simulink model "Bands7"  (R2018a)
settings: Solver=VariableStepAuto  StartTime=0.0  StopTime=0.01  RelTol=1e-3
undefined symbols (not defined in the file): fdesignblkfcn, G1, G2, G3, G4, G5, G6, G7, gcbh, get, T
libraries: dspsrcs4 x1, dspxfrm3 x1, dspobslib x1
(part 2 of 2)

== system Bands7/Filter Bank /Filter 5/Bandpass Filter ==
  In : Inport
  Generated Filter Block : DiscreteFir  Tag=BlockMethodSubSystem  Coefficients=[-9.58810852628409285e-08 2.32469628864830344e-08 3.86331465938965734e-07 -2.20783986023813804e-07 -1.02462161503425407e-06 9.81333351400442442e-07 2.09273408766862915e-06 -2.99371791475398828e-06 -3.31281199519531041e-06 7.28320341319092757e-06 3.72929278978732815e-06 -1.49118446680737189e-05 -1.28619054933032843e-06 2.64214782842553472e-05 -7.30535670538733667e-06 -4.08493754482887252e-05 2.62667010178946821e-05 5.4651471910311571e-05 -5.96059803468716439e-05 -6.08337254930435011e-05 0.000109152576803881542 4.90187993245668399e-05 -0.000171933793088775759 -6.98038786418440514e-06 0.000237712052040973639 -7.59195682598169175e-05 -0.000287739272451213301 0.000203714911831559986 0.000296061060386466359 -0.000368252612607931462 -0.000234224563044999241 0.000544966882564411012 7.94391823291172952e-05 -0.00069222980331757071 0.000175205090693047257 0.000756247105877000457 -0.000511177528820865924 -0.000682132059832164729 0.000879298715976650617 0.00042983022356125677 -0.00120235702500859549 8.77258524748186861e-06 0.00138752650373489021 -0.000596894132180304077 -0.00134769224831745205 0.00124972900223505501 0.00102741325130498683 -0.0018450930927680631 -0.000426327883119624086 0.00224817141909955257 -0.000388265080104680969 -0.00234590175869130949 0.00128635614321425968 0.00208214833483658449 -0.00209999739478021388 -0.00148249332143122895 0.00266396553918874521 0.000658647814734803546 -0.0028621525400130258 0.000212571742469404041 0.00266565875454846581 -0.000932999179653695786 -0.00214891728562074773 0.00133869642330399418 0.00147548828221558321 -0.00135067415892670063 -0.000854323950252250516 0.00100334938926574307 0.000477639688396269972 -0.000438719852644414991 -0.000459364165537671273 -0.000135265007016807301 0.000795224263203351232 0.000511214154350564083 -0.00136021337647840757 -0.000552719534013464326 0.00194748907395814056 0.000244187828567926819 -0.0023381878098927408 0.000299325687265161473 0.00237938988911029405 -0.000868808805288787903 -0.00204242142605657283 0.0012343976650798815 0.00143859817648006919 -0.00123031874608327089 -0.000783583969776330009 0.000820608820089682158 0.000320294511549712685 -0.000119378067820387741 -0.000226912149951525547 -0.000645229133491009355 0.00054439148237206338 0.00121327377293990388 -0.00115291167291446022 -0.00139256890304183235 0.00180982511450054396 0.00113764827880715857 -0.00223837184131480587 -0.00057554151761311117 0.00223549082946571023 -3.55594176082287081e-05 -0.0017570589557428162 0.000402862505289366588 0.00094481050398365421 -0.000315786849809520146 -8.00104639647764167e-05 -0.000262766749808934395 -0.000522506120992502206 0.00116955629342665774 0.000641039770527101907 -0.00209410080355902986 -0.000244184882697611556 0.00269575985622459886 -0.00048354262887346372 -0.00274133288650026249 0.00120335824971491267 0.00220797402718195517 -0.00155208512671623812 -0.00130634747033972379 0.00129152120570901786 0.000408549969613740665 -0.000416756600865931181 9.63079154092008047e-05 -0.000824671648667552309 3.58971676916477979e-05 0.00201744477211146089 -0.000791022589177617667 -0.00273938836172095673 0.00188315780959731355 0.00273707559579800235 -0.0028541270193768193 -0.00204361222754109468 0.00325286164607629588 0.000984752531566890094 -0.00282539339163617124 -6.22419908126786367e-05 0.00163636370351811513 -0.000245917406323728201 -6.56109702094782041e-05 -0.000309518401274032503 -0.00132835771435360172 0.00162485623429833338 0.00203067801396696491 -0.0032588688544591439 -0.00179094446626814697 0.00459217285623882837 0.000749014096506475657 -0.00507444040028377265 0.000594910613330368841 0.00446169817889733016 -0.00156551695937931826 -0.00294241174567129058 0.00158671475322137625 0.00109010796687163819 -0.000435806868879273497 0.000351161615849820692 -0.00163196222838977501 -0.000770829630763538625 0.00395176925736859426 -3.65997272116294625e-05 -0.00569705335793176636 0.00175038724886792969 0.00621616447243216168 -0.00361658993859075278 -0.00532206879955934506 ...(+7256 chars)]  InputProcessing=Columns as channels (frame based)
  Out : Outport
  wires:
  In/1 -> Generated Filter Block/1
  Generated Filter Block/1 -> Out/1

== system Bands7/Filter Bank /Filter 6/Bandpass Filter ==
  In : Inport
  Generated Filter Block : DiscreteFir  Tag=BlockMethodSubSystem  Coefficients=[-1.25255425151606446e-08 8.89638015557058461e-08 -1.00660481106791294e-07 -1.71542671618598763e-07 6.30727136722890552e-07 -4.94305586397416649e-07 -9.41860206286260817e-07 2.60648097200518803e-06 -1.51970142506445499e-06 -3.61925681579796005e-06 8.08811319906721527e-06 -3.49175116371090348e-06 -1.1058199124682812e-05 2.07298720252032752e-05 -6.26700739889994989e-06 -2.85833947368600613e-05 4.60081150553439048e-05 -8.46255439469102264e-06 -6.47651134006119471e-05 9.08836717492770435e-05 -6.44304383480617838e-06 -0.000131551007649326689 0.000162606489555876152 6.55019497498123363e-06 -0.000243150366983025702 0.000266628220200327355 4.05016863016043638e-05 -0.000413219537460888012 0.000404005983186840568 0.000107245375651426463 -0.000650375926198663683 0.000569142137305933137 0.000217148960754739669 -0.000952823316571735509 0.000748983248379460603 0.000374063015006662199 -0.00130367733422708963 0.000924651889340564049 0.000569711908969014187 -0.0016690706978893272 0.0010757723946409213 0.000779654225631718021 -0.0020009071412763371 0.00118658168412516052 0.000963374337522111194 -0.00224501117923517042 0.00125168654002985342 0.00107051093343472491 -0.00235353362539772676 0.00127864765455265052 0.00105348573675424209 -0.00229839700906786775 0.00128502102379148648 0.000884170524456743428 -0.00208118317329354348 0.00128930827508344026 0.000569581531915105055 -0.00173504472049494348 0.00129809096601209042 0.000160128275453357385 -0.0013163778185779477 0.00129442636713676066 -0.000255230684431742301 -0.000887736683498474154 0.0012339617878048127 -0.000569037034882513863 -0.000497533514369441661 0.00105396961220826767 -0.000687144670000418745 -0.000164654397395709356 0.000696271248643948572 -0.000563114550348206328 0.000124381414706665398 0.000138793139474224417 -0.000222564241775814856 0.000402274804298624654 -0.000575438119759497514 0.000234173942960876763 0.000695220164874023913 -0.00132582263997436381 0.000656595694415445445 0.000994957172509963652 -0.00192951581988383587 0.000891392271430931082 0.00124270486712862917 -0.0021872833289222687 0.000838066093421750095 0.00133698387209448617 -0.00195034211773934289 0.00049208229542788758 0.00116886917199326827 -0.00118712198309475531 -4.36832686119950414e-05 0.000675775510236198873 -2.33780320881614893e-05 -0.000588463769513059725 -0.000106648029153674808 0.00126649799565767924 -0.00094761156855736493 -0.00101986869618016056 0.00232436604491836115 -0.000988986407521479744 -0.00180479178356737335 0.00281579117468175495 -0.000701033724786980102 -0.00217461527176102034 0.00254679724689644074 -0.000205406431489680267 -0.00192000261778797233 0.001547055390059544 0.000286879953691100567 -0.00100959420040403879 8.29877302137138059e-05 0.000563205331859186072 0.000357732325524895325 -0.00141337049324328492 0.000506929173796110354 0.00178133273153402872 -0.00248238814787841468 0.000161355705397175963 0.00277292942611897294 -0.00279563684280270458 -0.000274283410010269879 0.00292624372174007724 -0.00227599204602179283 -0.000524851700467135474 0.00208324750860265986 -0.00112926975961976988 -0.000369102106795455838 0.000429435990301485981 0.000230803374986378014 0.000234616266742058391 -0.00153103119635096736 0.00134002527324787951 0.00108771505910517275 -0.00312742176945925415 0.00186306560293446419 0.00179669797102248734 -0.00375762732904636734 0.0017207113018726575 0.00192291441496002008 -0.00312251791732995982 0.00110854855834140132 0.00118620453962551154 -0.00136567096774006715 0.000394691550530183147 -0.000362156200121252611 0.000947076736786452091 -6.2252895142800825e-05 -0.00228292336609010622 0.00301487564500350436 -9.39968850170036242e-05 -0.00385680117783793576 0.00409449836575851833 0.000185135683972981641 -0.00433923981716520957 0.00378791711847140285 0.00042787366075095856 -0.00327610002517882571 0.00220736223664322849 0.000236086578017572434 -0.000753033868313336663 -5.73639565389522256e-05 -0.00060043166924552457 0.00254007828127078474 -0.00216656740971749983 ...(+7574 chars)]  InputProcessing=Columns as channels (frame based)
  Out : Outport
  wires:
  In/1 -> Generated Filter Block/1
  Generated Filter Block/1 -> Out/1

== system Bands7/Filter Bank /Filter 7/Bandpass Filter ==
  In : Inport
  Generated Filter Block : DiscreteFir  Tag=BlockMethodSubSystem  Coefficients=[1.73785777638198983e-08 5.53307655928696029e-08 -5.93261075754201142e-07 2.39151425515476142e-06 -6.48513630922282161e-06 1.34076757534754531e-05 -2.19514778171459608e-05 2.81125292022978393e-05 -2.54304009207347507e-05 7.77160995119231591e-06 2.56750310283883588e-05 -6.55244886674400545e-05 9.14386871994476703e-05 -7.89702444068962492e-05 1.38106561454960583e-05 9.2552034041583223e-05 -0.00019629525836815153 0.000233415676447405279 -0.000151571874020526014 -5.08961033605654563e-05 0.000302055501472180805 -0.000471848438432888762 0.000431172103111375027 -0.00013241288464823484 -0.000333224596582850524 0.000746513510533375097 -0.00085427096542935448 0.000512480179939020768 0.000197510427006736689 -0.000959758201500983009 0.00135473207975177678 -0.00108359599993431929 0.000169250182968863172 0.000993633909920033694 -0.00180012155352935171 0.00174972795567223316 -0.000751315472308702144 -0.000766187274657077343 0.00203186156748269 -0.00233241466939168932 0.00142321842761948514 0.000291081180231042168 -0.00193517820613313862 0.00262602239500718537 -0.00196835723958645008 0.000293868990911298408 0.00150845272728697389 -0.0024852883415886237 0.00215273227444568761 -0.000756876413467958624 -0.000891938083042786187 0.00190628271659362019 -0.00183031596807723611 0.000862643649298146676 0.000327866679015471245 -0.00105468168057194192 0.00103147230684341598 -0.000489843870350350065 -5.64931621242188649e-05 0.000213617305723943894 1.72764658636022303e-05 -0.000282287045395235141 0.000191187830209303781 0.000337066938522989266 -0.000967262286493930775 0.00117274045159026195 -0.000638002009766541018 -0.000456736720587986537 0.00149346411687726146 -0.00180136208817459689 0.00111384214709183229 0.00022266930227241171 -0.00144606237879843827 0.00185937487793159635 -0.00127182708650395689 0.00010099343590555876 0.000927702753756564952 -0.00126771357456859578 0.000882899855459425877 -0.000202374641937274371 -0.000245959001680188941 0.000236766286378755063 1.84297554528804847e-05 -9.55506433322579271e-05 -0.000245863515512851781 0.000816648406742686087 -0.00111117086353168353 0.000708953472085430223 0.00034094502674978809 -0.00146532583704598002 0.00191821712437509383 -0.00130563681239794101 -9.71264701631104212e-05 0.00148428656659214519 -0.00203795415744566742 0.00146868967293493414 -0.000195200415270114575 -0.000963955998027888261 0.00136091229557249978 -0.000936793425732064945 0.00019137900487701894 0.000253559263096094271 -0.000149852127253511915 -0.000209131820615096939 0.000275671817235847581 0.000243535178872410988 -0.00107401515967550805 0.00152992885853929332 -0.00104720483130511712 -0.000311250568527047329 0.00179069894225318852 -0.00241525031135572622 0.00167806708084373957 5.55323736112983416e-05 -0.00175082593289593901 0.00239166498988291776 -0.0016672764950968449 0.000160039317809309662 0.00110147822324460696 -0.00138960909861458653 0.000766756917958549508 4.33033260376633949e-05 -0.000287275888668670311 -0.000187283678973891571 0.000808814878002087631 -0.000774496991803525544 -0.000226394612659272586 0.00164800222324379105 -0.00241346232819209666 0.0017252554326152626 0.000248780409129921497 -0.00236902918372575329 0.00325960699621913362 -0.00227850033026366899 7.08292004378608337e-06 0.00212560423329483626 -0.00283152591795067477 0.00184713131904854638 -6.06991164213552861e-05 -0.00120412320246320124 0.00119731743223102987 -0.000268455396196960023 -0.000493372326332344887 0.000215848544903612829 0.000972748270827387268 -0.00198307593919396169 0.00163728073432557763 0.00029231390922890353 -0.00272181684798255587 0.00392778913270365546 -0.00280942033847018328 -0.000200142523385716815 0.00330432722784891391 -0.00453691107815650408 0.00313656089975522002 -8.76415400087590055e-05 -0.00259089078962688318 0.0032938420297948987 -0.00193793069632151307 -9.75114624074442123e-05 0.00113463438914623263 -0.000548396786190368489 -0.000765640550850884703 0.00119125222726294529 0.000166617635988841974 -0.00256879197647234521 ...(+7498 chars)]  InputProcessing=Columns as channels (frame based)
  Out : Outport
  wires:
  In/1 -> Generated Filter Block/1
  Generated Filter Block/1 -> Out/1
